simulink model "ColdStorage_PV_Thermal_ESS"  (R2020b)
settings: Solver=VariableStepAuto  StartTime=0.0  StopTime=8759  RelTol=1e-3
libraries: simulink x1
settings Model: SimulationMode=accelerator  Creator=jkarenzi  LastModifiedBy=michelechamberlin
settings SFSimCC: CustomCodeUndefinedFunction=UseInterfaceOnly

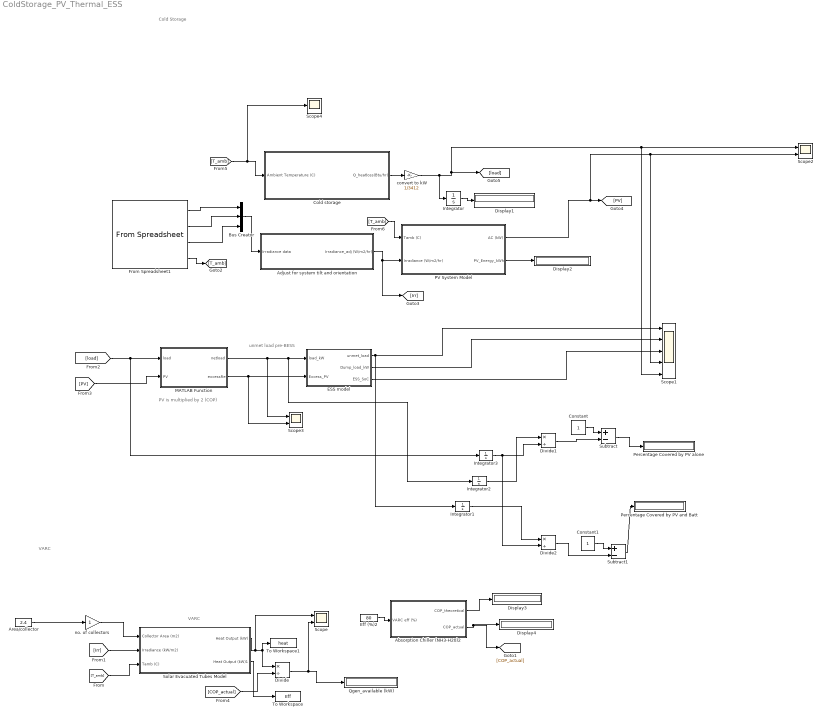
== system ColdStorage_PV_Thermal_ESS ==
  note: Cold Storage
  note: unmet load pre-BESS
  note: PV is multiplied by 2 (COP)
  note: VARC
  note: VARC
  Absorption Chiller (NH3-H20)2 : Subsystem  mask{Tgen=90, Tevap=-12, Tcond=40}
      mask prompts: Tgen "Generator Temperature (C)"; Tevap "Evaporator Temperature (C)"; Tcond "Condensor Temperature (C)"
      mask init:
      | %Initialize the generator, evaporator, and condensor temperature for the 
      | %NH3-H20 absorption chiller
      | 
      | TG = Tgen; %generator temperature
      | TE = Tevap; %evaporator temperature
      | TC = Tcond; %condensor temperature
  Adjust for system tilt and orientation : Subsystem  TreatAsAtomicUnit=on  mask{P1=65, P2=65, P3=180}
      mask prompts: P1 "Latitude (degrees)"; P2 "System tilt (degrees)"; P3 "System Orientation (degrees)"
      mask init:
      | L = P1;
      | B = P2;
      | Z = P3;
  Area/collector : Constant  Value=2.4
  Bus Creator : BusCreator  Inputs=3
  Cold storage : Subsystem  mask{P1=10, P2=10, P3=100, P5=30, P16=50, P17=10, P4=23, P11=0.01, P6=20, P7=0.92, P8=0.44, P9=130, P15=27, P12=1, P13=50, P14=5}
      mask prompts: P1 "Wall length (ft)"; P2 "Wall width (ft)"; P3 "Wall height (ft)"; P5 "R Value"; P16 "Space Usage (%)"; P17 "Wall thickness (inches)"; P4 "cold storage temp (F)"; P11 "Air changes per hour"; P6 "Mass per ft3 (lbs/ft3)"; P7 "Specific heat capacity above freezing (Btu/lbm.F)"; P8 "Specific heat capacity below freezing (Btu/lbm.F)"; P9 "Latent heat of fusion (Btu/lb)"; P15 "Freezing temp (F)"; P12 "Number of people in the room"; P13 "Wattage of the lights"; P14 "Number of lights"
      mask init:
      | %initialize the variables for the cold room temp
      | 
      | length = P1; 
      | width = P2;
      | height = P3;
      | T_amb = P4;
      | Rvalue = P5;
      | air_changes = P11;
      | mass = P6;
      | C_below = P7;
      | C_above = P8;
      | T_freeze = P15;
      | h_latent = P9;
      | no_of_people = P12;
      | lights_wattage = P13;
      | no_of_lights = P14;
      | space = P16;
      | thickness = P17;
      mask DialogControl ParameterGroupVar Prompt: Cold storage room details
      mask DialogControl Container3 Prompt: Food Product details
      mask DialogControl Container5 Prompt: Miscellaneous
  Constant : Constant
  Constant1 : Constant
  Display{1..4} (4 alike) : Display
  Divide : Product  Inputs=*/
  Divide1 : Product  Inputs=*/
  Divide2 : Product  Inputs=*/
  ESS model : Subsystem  mask{P1=100, P2=100, P3=30, P4=90, P5=80}
      mask prompts: P1 "ESS Capacity"; P2 "Initial_SoC (%)"; P3 "Min_SoC (%)"; P4 "Max_SoC (%)"; P5 "Battery Efficieny (%)"
      mask init:
      | Bat_capacity = P1;
      | Init_SoC = P2;
      | min_SoC = P3;
      | max_SoC = P4;
      | bat_eff = P5;
  Eff (%)2 : Constant  Value=80
  From Spreadsheet1 : FromSpreadsheet  FileName=C:\Users\michelechamberlin\Desktop\MicroFEWs\MATLAB Simulink\Cold Storage\Cold Storage Data.xlsx  SheetName=TananaData  Range=A1:E8761  SampleTime=1
  Integrator{,1..3} (4 alike) : Integrator
  MATLAB Function : MATLAB Function  TreatAsAtomicUnit=on
  PV System Model : Subsystem  mask{DC=50, TC=-0.0037, MM=15, Inv=96}
      mask prompts: DC "DC system size (kW)"; TC "Temp coeff (%)"; MM "System losses (%)"; Inv "Inverter efficiency (%)"
      mask init:
      | %initiliaze the parameters
      | %PV System size
      | DC_kW = DC; %DC system size
      | T_coeff = TC; %temp coefficient
      | 
      | %define losses
      | L_modules = MM; %losses due to module mismatch
      | %L_dirt = LD; %Losses due to dirt
      | 
      | inv_eff = Inv; %inverter efficiency
  Percentage Covered by PV alone : Display
  Percentage Covered by PV and Batt : Display
  Qgen_available (kW) : Display
  Scope : Scope  NumInputPorts=2
  Scope1 : Scope  NumInputPorts=5
  Scope2 : Scope  NumInputPorts=2
  Scope3 : Scope  NumInputPorts=2
  Scope4 : Scope
  Solar Evacuated Tubes Model : Subsystem
  Subtract : Sum  Inputs=+-
  Subtract1 : Sum  Inputs=+-
  To Workspace : ToWorkspace  VariableName=Eff  SampleTime=1
  To Workspace1 : ToWorkspace  VariableName=heat  SampleTime=1
  convert to kW : Gain  Gain=1/3412
  no. of collectors : Gain
  wires:
  Cold storage/1(Q_heatloss(Btu/hr)) -> convert to kW/1
  MATLAB Function/1(netload) -> Scope3/1, Integrator2/1, ESS model/1(load_kW)
  MATLAB Function/2(excessRe) -> Scope3/2, ESS model/2(Excess_PV)
  ESS model/1(unmet_load) -> Integrator1/1, Scope1/1
  [PV] -> MATLAB Function/2(PV)
  Absorption Chiller (NH3-H20)2/2(COP_actual) -> Display4/1, [COP_actual]
  Absorption Chiller (NH3-H20)2/1(COP_theoretical) -> Display3/1
  [T_amb] -> Solar Evacuated Tubes Model/3(Tamb (C))
  [Irr] -> Solar Evacuated Tubes Model/2(Irradiance (kW/m2))
  Solar Evacuated Tubes Model/1(Heat Output (kW)) -> Scope/1, Divide/1, To Workspace1/1
  Area/collector/1 -> no. of collectors/1
  no. of collectors/1 -> Solar Evacuated Tubes Model/1(Collector Area (m2))
  ESS model/2(Dump_load_kW) -> Scope1/2
  ESS model/3(ESS_SoC) -> Scope1/3
  Eff (%)2/1 -> Absorption Chiller (NH3-H20)2/1(VARC eff (%))
  Divide/1 -> Scope/2, Qgen_available (kW)/1
  From Spreadsheet1/3 -> Bus Creator/3
  PV System Model/1(AC (kW)) -> Scope2/2, Scope1/4, [PV]
  From Spreadsheet1/1 -> Bus Creator/1
  From Spreadsheet1/2 -> Bus Creator/2
  From Spreadsheet1/4 -> [T_amb]
  PV System Model/2(PV_Energy_kWh) -> Display2/1
  Bus Creator/1 -> Adjust for system tilt and orientation/1(Irradiance data)
  Adjust for system tilt and orientation/1(Irradiance_adj (W/m2/hr)) -> PV System Model/2(Irradiance (W/m2/hr)), [Irr]
  [T_amb] -> Scope4/1, Cold storage/1(Ambient Temperature (C))
  [COP_actual] -> Divide/2
  convert to kW/1 -> Integrator/1, Scope2/1, Scope1/5, [load]
  [load] -> Integrator3/1, MATLAB Function/1(load)
  [T_amb] -> PV System Model/1(Tamb (C))
  Integrator/1 -> Display1/1
  Solar Evacuated Tubes Model/2(Heat Output (kW)1) -> To Workspace/1
  Integrator3/1 -> Divide2/2, Divide1/2
  Integrator1/1 -> Divide2/1
  Integrator2/1 -> Divide1/1
  Constant/1 -> Subtract/1
  Constant1/1 -> Subtract1/1
  Divide1/1 -> Subtract/2
  Subtract/1 -> Percentage Covered by PV alone/1
  Divide2/1 -> Subtract1/2
  Subtract1/1 -> Percentage Covered by PV and Batt/1

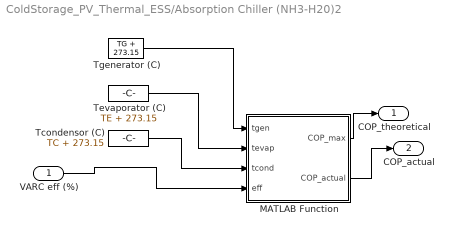
== system ColdStorage_PV_Thermal_ESS/Absorption Chiller (NH3-H20)2 ==
  VARC eff (%) : Inport
  MATLAB Function : MATLAB Function  TreatAsAtomicUnit=on
  Tcondensor (C) : Constant  Value=TC + 273.15
  Tevaporator (C) : Constant  Value=TE + 273.15
  Tgenerator (C) : Constant  Value=TG + 273.15
  COP_theoretical : Outport  VectorParamsAs1DForOutWhenUnconnected=off
  COP_actual : Outport  Port=2  VectorParamsAs1DForOutWhenUnconnected=off
  wires:
  Tcondensor (C)/1 -> MATLAB Function/3(tcond)
  Tevaporator (C)/1 -> MATLAB Function/2(tevap)
  Tgenerator (C)/1 -> MATLAB Function/1(tgen)
  MATLAB Function/1(COP_max) -> COP_theoretical/1
  MATLAB Function/2(COP_actual) -> COP_actual/1
  VARC eff (%)/1 -> MATLAB Function/4(eff)

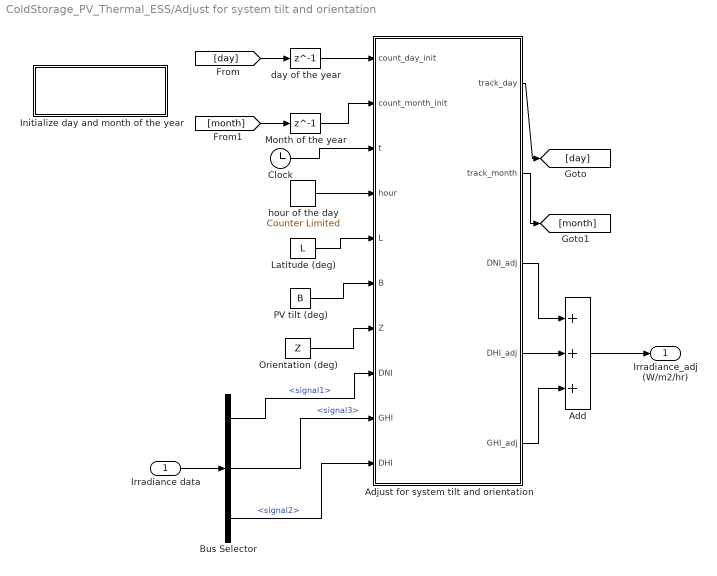
== system ColdStorage_PV_Thermal_ESS/Adjust for system tilt and orientation ==
  Irradiance data : Inport
  Add : Sum  Inputs=+++
  Adjust for system tilt and orientation : MATLAB Function  TreatAsAtomicUnit=on
  Bus Selector : BusSelector  OutputSignals=signal1,signal3,signal2
  Clock : Clock
  Initialize day and month of the year : Subsystem  TreatAsAtomicUnit=on
  Latitude (deg) : Constant  Value=L
  Month of the year : Delay  DelayLength=1  InitialCondition=0  SampleTime=1
  Orientation (deg) : Constant  Value=Z
  PV tilt (deg) : Constant  Value=B
  day of the year : Delay  DelayLength=1  InitialCondition=0  SampleTime=1
  hour of the day : simulink/Sources/Counter Limited  uplimit=24  tsamp=1
  Irradiance_adj (W/m2/hr) : Outport
  wires:
  [month] -> Month of the year/1
  Adjust for system tilt and orientation/1(track_day) -> [day]
  Adjust for system tilt and orientation/5(GHI_adj) -> Add/3
  day of the year/1 -> Adjust for system tilt and orientation/1(count_day_init)
  PV tilt (deg)/1 -> Adjust for system tilt and orientation/6(B)
  Month of the year/1 -> Adjust for system tilt and orientation/2(count_month_init)
  Adjust for system tilt and orientation/2(track_month) -> [month]
  hour of the day/1 -> Adjust for system tilt and orientation/4(hour)
  Clock/1 -> Adjust for system tilt and orientation/3(t)
  [day] -> day of the year/1
  Orientation (deg)/1 -> Adjust for system tilt and orientation/7(Z)
  Adjust for system tilt and orientation/3(DNI_adj) -> Add/1
  Adjust for system tilt and orientation/4(DHI_adj) -> Add/2
  Latitude (deg)/1 -> Adjust for system tilt and orientation/5(L)
  Add/1 -> Irradiance_adj (W/m2/hr)/1
  Irradiance data/1 -> Bus Selector/1
  Bus Selector/1 -> Adjust for system tilt and orientation/8(DNI)  "<signal1>"
  Bus Selector/2 -> Adjust for system tilt and orientation/9(GHI)  "<signal3>"
  Bus Selector/3 -> Adjust for system tilt and orientation/10(DHI)  "<signal2>"

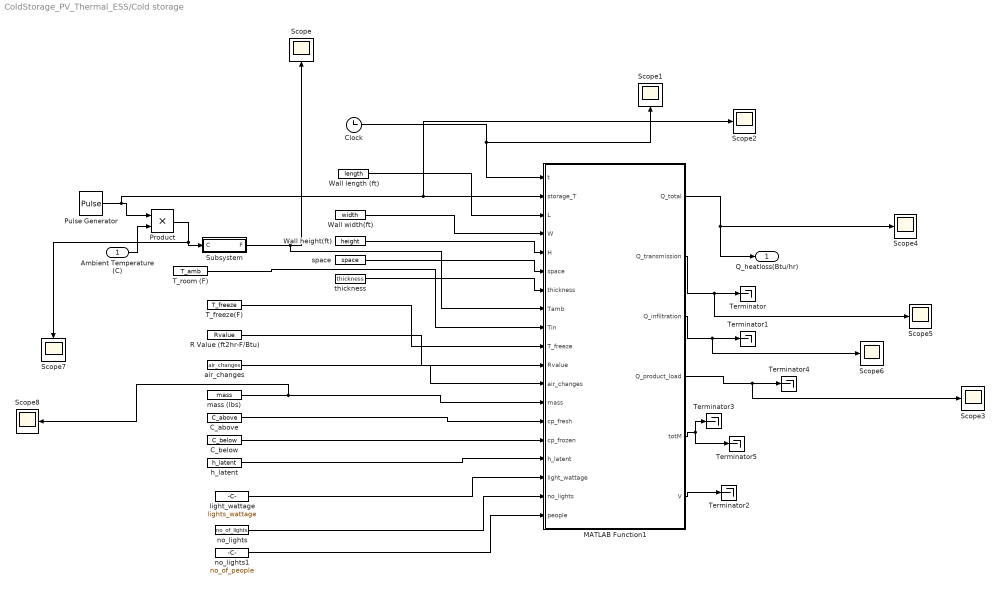
== system ColdStorage_PV_Thermal_ESS/Cold storage ==
  Ambient Temperature (C) : Inport
  C_above : Constant  Value=C_above
  C_below : Constant  Value=C_below
  Clock : Clock
  MATLAB Function1 : MATLAB Function  TreatAsAtomicUnit=on
  Product : Product
  Pulse Generator : DiscretePulseGenerator  PulseType=Time based  Period=24  PulseWidth=42  PhaseDelay=8
  R Value (ft2hr-F/Btu) : Constant  Value=Rvalue
  Scope{,1..8} (9 alike) : Scope
  Subsystem : Subsystem
  T_freeze(F) : Constant  Value=T_freeze
  T_room (F) : Constant  Value=T_amb
  Terminator{,1..5} (6 alike) : Terminator
  Wall height(ft) : Constant  Value=height
  Wall length (ft) : Constant  Value=length
  Wall width(ft) : Constant  Value=width
  air_changes : Constant  Value=air_changes
  h_latent : Constant  Value=h_latent
  light_wattage : Constant  Value=lights_wattage
  mass (lbs) : Constant  Value=mass
  no_lights : Constant  Value=no_of_lights
  no_lights1 : Constant  Value=no_of_people
  space : Constant  Value=space
  thickness : Constant  Value=thickness
  Q_heatloss(Btu/hr) : Outport  VectorParamsAs1DForOutWhenUnconnected=off
  wires:
  R Value (ft2hr-F/Btu)/1 -> MATLAB Function1/11(Rvalue)
  MATLAB Function1/1(Q_total) -> Scope4/1, Q_heatloss(Btu/hr)/1
  Wall length (ft)/1 -> MATLAB Function1/3(L)
  T_room (F)/1 -> MATLAB Function1/9(Tin)
  Ambient Temperature (C)/1 -> Product/2
  Wall width(ft)/1 -> MATLAB Function1/4(W)
  Wall height(ft)/1 -> MATLAB Function1/5(H)
  T_freeze(F)/1 -> MATLAB Function1/10(T_freeze)
  air_changes/1 -> MATLAB Function1/12(air_changes)
  mass (lbs)/1 -> Scope8/1, MATLAB Function1/13(mass)
  C_below/1 -> MATLAB Function1/15(cp_frozen)
  C_above/1 -> MATLAB Function1/14(cp_fresh)
  h_latent/1 -> MATLAB Function1/16(h_latent)
  Subsystem/1(F) -> Scope/1, MATLAB Function1/8(Tamb)
  light_wattage/1 -> MATLAB Function1/17(light_wattage)
  no_lights/1 -> MATLAB Function1/18(no_lights)
  no_lights1/1 -> MATLAB Function1/19(people)
  MATLAB Function1/2(Q_transmission) -> Scope5/1, Terminator/1
  MATLAB Function1/3(Q_infiltration) -> Scope6/1, Terminator1/1
  space/1 -> MATLAB Function1/6(space)
  thickness/1 -> MATLAB Function1/7(thickness)
  Clock/1 -> Scope1/1, MATLAB Function1/1(t)
  Product/1 -> Scope7/1, Subsystem/1(C)
  MATLAB Function1/4(Q_product_load) -> Scope3/1, Terminator4/1
  MATLAB Function1/6(V) -> Terminator2/1
  MATLAB Function1/5(totM) -> Terminator3/1, Terminator5/1
  Pulse Generator/1 -> Scope2/1, MATLAB Function1/2(storage_T), Product/1

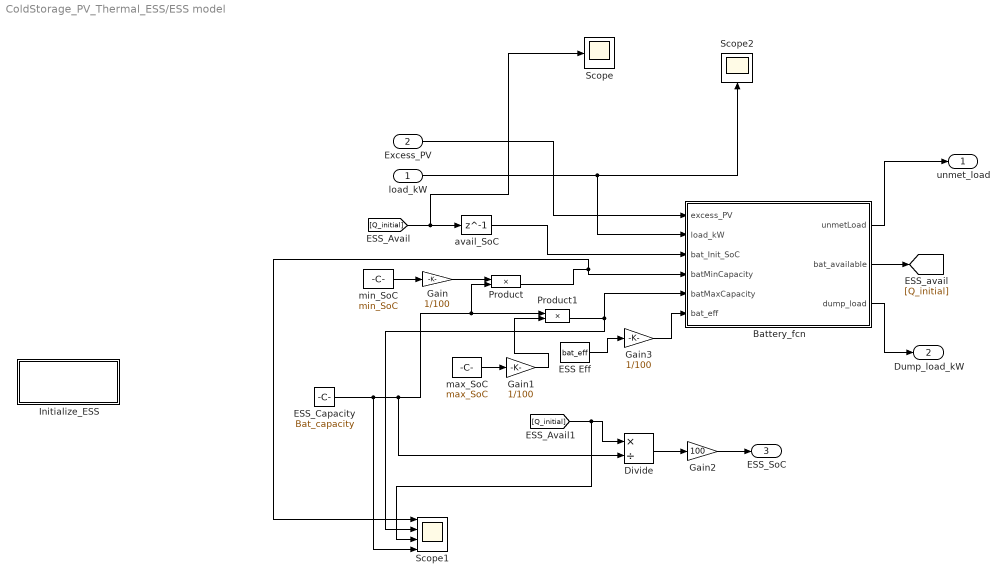
== system ColdStorage_PV_Thermal_ESS/ESS model ==
  load_kW : Inport
  Excess_PV : Inport  Port=2
  Battery_fcn : MATLAB Function  TreatAsAtomicUnit=on
  Divide : Product  Inputs=*/
  ESS Eff : Constant  Value=bat_eff
  "ESS_Capacity " : Constant  Value=Bat_capacity
  Gain : Gain  Gain=1/100
  Gain1 : Gain  Gain=1/100
  Gain2 : Gain  Gain=100
  Gain3 : Gain  Gain=1/100
  Initialize_ESS : Subsystem  TreatAsAtomicUnit=on
  Product : Product
  Product1 : Product
  Scope : Scope
  Scope1 : Scope  NumInputPorts=4
  Scope2 : Scope
  avail_SoC : Delay  DelayLength=1  InitialCondition=0  SampleTime=1
  max_SoC : Constant  Value=max_SoC
  min_SoC : Constant  Value=min_SoC
  unmet_load : Outport
  Dump_load_kW : Outport  Port=2
  ESS_SoC : Outport  Port=3
  wires:
  Excess_PV/1 -> Battery_fcn/1(excess_PV)
  avail_SoC/1 -> Battery_fcn/3(bat_Init_SoC)
  Battery_fcn/1(unmetLoad) -> unmet_load/1
  [Q_initial] -> Scope/1, avail_SoC/1
  max_SoC/1 -> Gain1/1
  min_SoC/1 -> Gain/1
  Gain/1 -> Product/1
  Product/1 -> Scope1/1, Battery_fcn/4(batMinCapacity)
  Product1/1 -> Scope1/2, Battery_fcn/5(batMaxCapacity)
  Gain1/1 -> Product1/2
  load_kW/1 -> Scope2/1, Battery_fcn/2(load_kW)
  Battery_fcn/2(bat_available) -> [Q_initial]
  Battery_fcn/3(dump_load) -> Dump_load_kW/1
  ESS Eff/1 -> Gain3/1
  Gain3/1 -> Battery_fcn/6(bat_eff)
  "ESS_Capacity "/1 -> Scope1/4, Divide/2, Product1/1, Product/2
  [Q_initial] -> Scope1/3, Divide/1
  Divide/1 -> Gain2/1
  Gain2/1 -> ESS_SoC/1

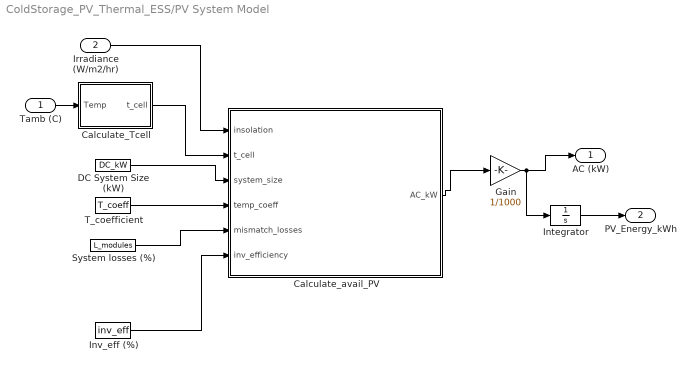
== system ColdStorage_PV_Thermal_ESS/PV System Model ==
  Tamb (C) : Inport
  Irradiance (W/m2/hr) : Inport  Port=2
  Calculate_Tcell : MATLAB Function  TreatAsAtomicUnit=on
  Calculate_avail_PV : MATLAB Function  TreatAsAtomicUnit=on
  DC System Size (kW) : Constant  Value=DC_kW
  Gain : Gain  Gain=1/1000
  Integrator : Integrator
  Inv_eff (%) : Constant  Value=inv_eff
  System losses (%) : Constant  Value=L_modules
  T_coefficient : Constant  Value=T_coeff
  AC (kW) : Outport  VectorParamsAs1DForOutWhenUnconnected=off
  PV_Energy_kWh : Outport  Port=2  VectorParamsAs1DForOutWhenUnconnected=off
  wires:
  Gain/1 -> AC (kW)/1, Integrator/1
  Integrator/1 -> PV_Energy_kWh/1
  Calculate_avail_PV/1(AC_kW) -> Gain/1
  Irradiance (W/m2/hr)/1 -> Calculate_avail_PV/1(insolation)
  Calculate_Tcell/1(t_cell) -> Calculate_avail_PV/2(t_cell)
  Tamb (C)/1 -> Calculate_Tcell/1(Temp)
  DC System Size (kW)/1 -> Calculate_avail_PV/3(system_size)
  T_coefficient/1 -> Calculate_avail_PV/4(temp_coeff)
  System losses (%)/1 -> Calculate_avail_PV/5(mismatch_losses)
  Inv_eff (%)/1 -> Calculate_avail_PV/6(inv_efficiency)

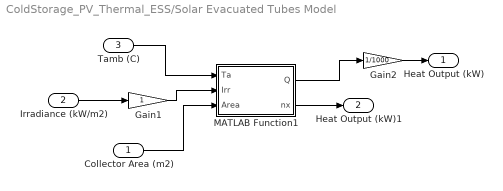
== system ColdStorage_PV_Thermal_ESS/Solar Evacuated Tubes Model ==
  Collector Area (m2) : Inport
  Irradiance (kW/m2) : Inport  Port=2
  Tamb (C) : Inport  Port=3
  Gain1 : Gain
  Gain2 : Gain  Gain=1/1000
  MATLAB Function1 : MATLAB Function  TreatAsAtomicUnit=on
  Heat Output (kW) : Outport  VectorParamsAs1DForOutWhenUnconnected=off
  Heat Output (kW)1 : Outport  Port=2  VectorParamsAs1DForOutWhenUnconnected=off
  wires:
  Tamb (C)/1 -> MATLAB Function1/1(Ta)
  Irradiance (kW/m2)/1 -> Gain1/1
  MATLAB Function1/1(Q) -> Gain2/1
  Gain1/1 -> MATLAB Function1/2(Irr)
  Collector Area (m2)/1 -> MATLAB Function1/3(Area)
  Gain2/1 -> Heat Output (kW)/1
  MATLAB Function1/2(nx) -> Heat Output (kW)1/1

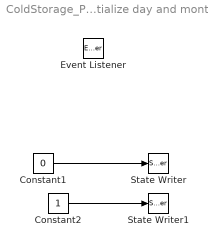
== system ColdStorage_PV_Thermal_ESS/Adjust for system tilt and orientation/Initialize day and month of the year ==
  Constant1 : Constant  Value=0
  Constant2 : Constant
  Event Listener : EventListener  DisableCoverage=on  EventName=reset
  State Writer : StateWriter  StateOwnerBlock=../../day of the year
  State Writer1 : StateWriter  StateOwnerBlock=../../Month of the year
  wires:
  Constant2/1 -> State Writer1/1
  Constant1/1 -> State Writer/1

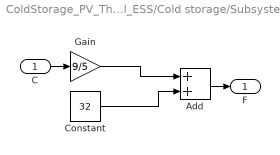
== system ColdStorage_PV_Thermal_ESS/Cold storage/Subsystem ==
  C : Inport
  Add : Sum
  Constant : Constant  Value=32
  Gain : Gain  Gain=9/5
  F : Outport
  wires:
  Constant/1 -> Add/2
  C/1 -> Gain/1
  Gain/1 -> Add/1
  Add/1 -> F/1

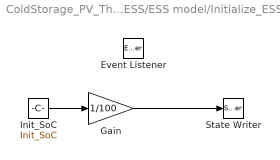
== system ColdStorage_PV_Thermal_ESS/ESS model/Initialize_ESS ==
  Event Listener : EventListener  DisableCoverage=on  EventName=reset
  Gain : Gain  Gain=1/100
  Init_SoC : Constant  Value=Init_SoC
  State Writer : StateWriter  StateOwnerBlock=../../avail_SoC
  wires:
  Init_SoC/1 -> Gain/1
  Gain/1 -> State Writer/1

== matlab function ColdStorage_PV_Thermal_ESS/Cold storage/MATLAB Function1 ==
  data: t input; storage_T input; L input; W input; H input; space input; thickness input; Tamb input; Tin input; T_freeze input; Q_total output; Rvalue input; air_changes input; mass input; cp_fresh input; cp_frozen input; h_latent input; light_wattage input; no_lights input; people input; Q_transmission output; Q_infiltration output; Q_product_load output; totM output; V output
function [Q_total,Q_transmission,Q_infiltration,Q_product_load,totM,V ] = fcn(t,storage_T,L,W,H,space,thickness, Tamb,Tin,T_freeze,Rvalue,air_changes, mass,cp_fresh,cp_frozen,h_latent,light_wattage,no_lights,people)
%function estimates the energy requirements of a community cold storage
%unit
%Assume Polyurethane foam is the insulator with a K value of 0.015
%Btu/(hr.ft.F)

%Uwall - Overall heat transfer of the walls, roof, floor
if (t>2000 && t<6000)
    if(Tamb<=0)
        deltaT = 0;
    end
end

deltaT = (Tamb-Tin); 
U = 1/Rvalue;
top_bottom_area = L*W*2; 
side_walls = L*H*4;
thickness = thickness/12; %convert to ft
V = (L-thickness)*(W-thickness)*(H-thickness);
%V = V * 0.0283168; %convert to cubic metres

%1. Transmission Load
Q_transmission = ((top_bottom_area*U*deltaT)+ (side_walls*U*deltaT));

% vroom = 0.78; %volume of dry air at RH of 95%
% mair = (V/vroom)*0.2; %mass flow rate
% hroom = 11; %kj/kg of fry air
% hambient = 93; 
% wambient = 0.024; %kg/kg of dry air (ambient)
% wroom = 0.0038; %kg/kg of dry air (room)
% hfg = 2466; %kj/kg heat of vaporization of water at avg. temp (15C)
% 
% %2. Air infiltration
% Q_inf_sensible =mair*(hambient-hroom);
% Q_inf_latent = (wambient - wroom)*mair*hfg;
% 
% Q_infiltration = (Q_inf_sensible + Q_inf_latent); %in kW

% V is ft3, air_changes is 1/hr, delta T is F, 
Q_infiltration = V*air_changes*deltaT*0.01838; % This was wrong, the units don't add up, the units....
%0.1838 was added, it results from air heat capacity 0.24 BTU/lb/F and air density of
%0.0765 lb/ft3
%3. product load
T_load = 68; % JK value 68, DS suggested 50
space = space/100;
Q_cooling_fresh = (space*V*mass)*cp_fresh*(T_load-T_freeze); % v volume, space is space usage in percentage
totM = (space*V*mass);
Q_freezing = (space*V*mass)*h_latent;
Q_cooling_frozen = (space*V*mass)*cp_frozen*(T_freeze-Tin);


%Q_product_load = ((Q_cooling_fresh + Q_freezing + Q_cooling_frozen)/(storage_T*24));%one-time calculation

%Assume a daily storage temp of 10 hrs
Q_product_load = ((Q_cooling_fresh + Q_freezing + Q_cooling_frozen)/(10)/90);%one-time calculation 
%division by 10 is for the 10 operational hours in one day.
%Change here by MJC: Division by 90 is the number of days the product stays
%in the cooler (assuming 3 months average residence time in cooler), otherwise the product cooling load gets calculated as if
%new product is added every day... which might be the case for industrial
%fishprocessing coolers, but not for residential coolers!

if(storage_T<=0)
  Q_product_load =  0;
  
end


% if(mod(t,storage_T*24)==0)
% Q_product_load = Q_product_load/(storage_T*24);
% end

if(Tamb <= Tin)
  Q_product_load = 0;
end

%4. Q_miscellaneous
%4.1 people
Q_people = (270 - 6*Tin)*people; %in watts
Q_lights = light_wattage*no_lights; %in watts
Q_miscellaneous = Q_people+Q_lights;

%5. Total heat load
Q_total = 1.1*(Q_transmission + Q_infiltration + Q_miscellaneous + Q_product_load );
%Q_total = (Q_transmission + Q_infiltration + Q_miscellaneous);

if(Q_total<0)
    Q_total = 0;
end

== matlab function ColdStorage_PV_Thermal_ESS/Solar Evacuated Tubes Model/MATLAB Function1 ==
  data: Ta input; Q output; Irr input; Area input; nx output
function [Q,nx] = fcn(Ta,Irr,Area)

no = 0.845; a1 = 1.47; a2 = 0.01; %units for a1, and a2 are W/(k2.m2)
Tm = 70; %avg temp at the inlet-outlet water temp

x = (Tm - Ta)/Irr;
nx = no - a1*x - a2*Irr*x^2;
if(nx<0)
    nx = 0;
end
Q = Area * Irr * nx; %Area is the abosrber area

TF = isfinite(Q); %check if Q is nan

if(TF == 0)
    Q = 0;
end

== matlab function ColdStorage_PV_Thermal_ESS/PV System Model/Calculate_Tcell ==
  data: Temp input; t_cell output
function t_cell  = T_cell(Temp)
%function reads the ambient temperature in deg. celcius and calculates the
%cell temperature
NOCT = 47; %Nominal Operating Cell Temperature
A_Temp = 20; %Ambient Temperature under NOCT
Solar_Irr = 0.8; %Solar Irrandiance of 0.8kW/m2
t_cell = Temp + ((NOCT-A_Temp)/Solar_Irr)*1; %Estimating Cell Temperature at 1-sun

== matlab function ColdStorage_PV_Thermal_ESS/PV System Model/Calculate_avail_PV ==
  data: insolation input; AC_kW output; t_cell input; system_size input; temp_coeff input; mismatch_losses input; inv_efficiency input
function AC_kW = Solar_PV(insolation,t_cell,system_size, temp_coeff, mismatch_losses,inv_efficiency)

%function approximates the DC, AC, and energy (Kwh) solar PV Output using the
%peak sun hours approach as outlined in the Gilbert M. Masters 'Renewable and
%Efficient Electric Power Systems'.
%tcell: cell temperature
%system_size: DC kW system size
%insolation: kWh/m2/day or (hrs/day) of full sun available


if (insolation<0) %Check for insolation/Irradiance value is less than zero
    insolation = 0; 
end
DC_Power_kW = insolation*system_size *(1-temp_coeff*(t_cell-25));
%DC_Power_kW = system_size*(1-temp_coeff*(t_cell-25)); % Calculate DC Power using the new cell temperature
AC_kW = DC_Power_kW*(1-(mismatch_losses/100))*(inv_efficiency/100); %calculate AC Power accounting for losses


%kWh_output_AC = AC_kW *insolation; %hrs/day of full sun using the peak-sun hours
%PV_kWh = kWh_output_AC;
%PV_kWh = kWh_output_AC * 30; %monthly Output (Assume 30 days for 1 full month)

== matlab function ColdStorage_PV_Thermal_ESS/MATLAB Function ==
  data: load input; netload output; PV input; excessRe output
function [netload,excessRe] = fcn(load,PV)
Re = (2)*PV; %Available renewable energy, assume a COP of 2
if(Re>load)
    netload = 0;
    excessRe = Re-load;
elseif(Re<=load)
    netload = load-Re;
    excessRe = 0;
else
    netload = 0;
    excessRe = 0;
end

== matlab function ColdStorage_PV_Thermal_ESS/Adjust for system tilt and orientation/Adjust for system tilt and orientation ==
  data: track_day output; track_month output; count_day_init input; count_month_init input; t input; hour input; L input; B input; Z input; DNI input; DNI_adj output; DHI_adj output; GHI input; DHI input; GHI_adj output
function [track_day, track_month, DNI_adj,DHI_adj,GHI_adj] = fcn(count_day_init,count_month_init,t,hour,L,B,Z,DNI,GHI,DHI)

%L: Latitude
%B: tilt
%Z: surface azimuth
hour = double(hour);

m=[0 31 59 90 120 151 181 212 243 273 304 334]; %days in the year

if (mod(t,24) ==0)
track_day = count_day_init + 1;
else
  track_day = count_day_init; 
end

if(mod(t,730) == 0)
 track_month = count_month_init + 1;
else
    track_month = count_month_init;
end

n= m(track_month)+ track_day;

%declination angle
declination_angle = 23.45*sin(360*(284+n)/365*pi/180); %see equ(1)   
d=declination_angle*pi/180; 

%hour angle
hour_angle = (hour-12)*15; %see equ(2)      
h=hour_angle*pi/180; 

%altitude angle
Altitude_angle = asin(sin(L)*sin(d)+cos(L)*cos(d)*cos(h))*180/pi; %see equ(3)
a=Altitude_angle*pi/180;

Solar_zenith_angle = 90-Altitude_angle;

phi =Solar_zenith_angle*pi/180; 
Solar_azimuth_angle= asin(cos(d)*sin(h)/cos(a))*180/pi; %see equ(4)
z =Solar_azimuth_angle*pi/180; 
 
L = L*180/pi;
Z = Z*180/pi;
B = B*180/pi;

Incidence_angle = acos(sin(L)*sin(d)*cos(B)- cos(L)*sin(d)*sin(B)*cos(Z)+ cos(L)*cos(d)*cos(h)*cos(B)...
+ sin(L)*cos(d)*cos(h)*sin(B)*cos(Z)+cos(d) *sin(h)*sin(B)*sin(Z))*180/pi; %see equ(5) 
theta =Incidence_angle*pi/180; 
%RB=cos(theta)/cos(phi); %see equ(6) 
HSRC = [ acos(complex((-tan(L)*tan(d)))) acos(complex((-tan(L-B)*tan(d))))];
HSRC = min(HSRC);
RB = (cos(L-B)*cos(d)*sin(HSRC) + HSRC*sin(L-B)*sin(d)) /(cos(L)*cos(d)*sin(HSRC) + HSRC*sin(L)*sin(d));
    
DNI_adj = abs(cos(theta))*DNI;
DHI_adj = (1+cos(B))/2*DHI;
GHI_adj = (1-cos(B))/2 * GHI;


end

== matlab function ColdStorage_PV_Thermal_ESS/ESS model/Battery_fcn ==
  data: excess_PV input; unmetLoad output; load_kW input; bat_Init_SoC input; batMinCapacity input; batMaxCapacity input; bat_eff input; bat_available output; dump_load output
function [ unmetLoad,bat_available,dump_load] = batt_fcn(excess_PV,load_kW,bat_Init_SoC,batMinCapacity,batMaxCapacity,bat_eff)
%if generation meets demand, no unmentload, energy storage unchanged, no
 %excess renewable
 %Here load_kW represents unmet load 
bat_available = bat_Init_SoC; %%MJC: this is not SOC, this is tot available energy capacity
%if load is greater than generation, use battery to cover the unmet load     
if(load_kW > 0)%MJC: automatically means there is no PV generation, because load here, is unmet load from previous functions
    %Check how much energy the battery has. If at minimum, send unmet
    %load to diesel
    if(bat_available <= batMinCapacity)
        %fprintf(2,'Battery was below Min_Cap')
        
        bat_available = batMinCapacity; % MJC: erase this line, it corrects future error and gifts cap to BESS
        unmetLoad = load_kW;
        dump_load = 0 ;
        
        
        %If there's power in the battery, meet the load till the minimum is reached. then send
        %rest to the diesel
    elseif((bat_available > batMinCapacity)&& (load_kW>(bat_available-batMinCapacity))) %batt avail greater bat min cap
        %  if(load_kW>(bat_available-batMinCapacity)) %unmet load > avail battery
        %fprintf(2,'Battery used')
        
        bat_available = batMinCapacity;
        unmetLoad = load_kW - (bat_Init_SoC - batMinCapacity); %MJC replace bat_init_ with Bat_available
        dump_load = 0 ;
        
        
        %neglect self discharge rate
    elseif((bat_available > batMinCapacity)&& (load_kW<=(bat_available-batMinCapacity)))
        
        bat_available = bat_Init_SoC - load_kW;
        unmetLoad = 0;
        dump_load = 0;
        

        
    else %if(bat_available>=batMinCapacity) %Numeric weirdness, never hits this case, but Matlab requires it...?
        fprintf(2,'Battery ')
        bat_available = bat_Init_SoC;
        unmetLoad = 0;
        dump_load = 0;
        
    end
    % end
    %if generation meets demand and there's no excess PV
elseif ((load_kW == 0)&& (excess_PV ==0))
    bat_available =  bat_Init_SoC;
    unmetLoad = 0;
    dump_load = 0 ;
    %if there is excess PV, charge the ESS. Ignoring the self discharge rates
elseif(excess_PV >0) %automaticall load <=0
    
    %  PVExcess = P_charge_kW - load_kW;
    if((bat_available+excess_PV/bat_eff)>=batMaxCapacity)
        dump_load = excess_PV-((batMaxCapacity-bat_available)/(bat_eff));%%MJC line was: dump_load = excess_PV
        bat_available = batMaxCapacity;
        unmetLoad = 0;
    else
        bat_available =  bat_available + excess_PV *(bat_eff);
        unmetLoad = 0;
        dump_load = 0;
    end
    
    
    
else
    bat_available = bat_Init_SoC;
    unmetLoad = 0;
    dump_load = 0;
end
end

== matlab function ColdStorage_PV_Thermal_ESS/Absorption Chiller (NH3-H20)2/MATLAB Function ==
  data: tgen input; COP_max output; tevap input; tcond input; eff input; COP_actual output
function [COP_max,COP_actual] = fcn(tgen,tevap,tcond,eff)
%function estimates the maximum COP of the absorption chiller given the 
%working temperatures
%Qe: Cooling Load
%Qgen: Q available at the generator
COP_max = (1/((tcond/tevap)-1)) * (1-(tcond/tgen));
COP_actual = COP_max * (eff/100); %actual COP of the chiller given the efficiency
%Qe = COP_actual * Qgen;
%Qe = Qe * 3.517; %convert to kW

% Qgen = Qe/COP_actual; %heat input to the generator
% Qgen = 3.517*Qgen; %convert to kW
